simulink model "UAM_Flight_control"  (R2024b)
settings: Solver=FixedStepAuto  StartTime=0.0  StopTime=inf  RelTol=1e-3  EnableMultiTasking=on
undefined symbols (not defined in the file): CityMission, control, controlParams, ControlSampleTime, Cruise_a, DiscIntNeverNeededParam, Earth, FixedWingMission, flightState, FSState, FWControlParams, FWTrimSpeed, HoverMission, params, position, R_WAYPOINTTRANSITION, TransitionMission, uavParam, Vt, w_trim, WGS84, zGround
libraries: slpidlib x56, simulink x35, uavalgslib x8, robotcorelib x2, simulink_extras x2, mspfiltlib x1, aerolibtransform2 x1
(part 11 of 12)

== stateflow chart UAM_Flight_control/Flightmode/Manual/Basic Control  Switching ==
  state STATE_MACHINE
    state Althold
      en:
      flightMode = flightState.Hover;
      %Hover SP
      HoverSPBUS.X = NaN;
      HoverSPBUS.Y = NaN;
      HoverSPBUS.Z = pose(3);
      HoverSPBUS.Yaw = NaN;
    state Stablized
      en:
      flightMode = flightState.Hover;
      %Hover SP
      HoverSPBUS.X = NaN;
      HoverSPBUS.Y = NaN;
      HoverSPBUS.Z = NaN;
      HoverSPBUS.Yaw = NaN;
    state Transition
      en:
      flightMode = flightState.Transition;
      controlMode.inTransition = 1;
      controlMode.TransitionCondition = 0;
    state FWCOMPLETE
      en:
      controlMode.TransitionCondition=1;
      flightMode = flightState.FixedWing;
    state Loiter
      en:
      flightMode = flightState.Hover;
      %Hover SP
      HoverSPBUS.X = pose(1);
      HoverSPBUS.Y = pose(2);
      HoverSPBUS.Z = pose(3);
      HoverSPBUS.Yaw = NaN;
    state Start
      en:
      flightMode=PresetMode;
      %conrtolmode
      controlMode.lateralGuidance = 0;
      controlMode.airspeedAltitude = 0;
      controlMode.attitude = 0;
      controlMode.manual = 1;
      controlMode.armed = 0;
      controlMode.inTransition = 0;
      controlMode.TransitionCondition = 0;
      controlMode.BackTransitionCondition = 0;
      controlMode.land=1;
    state FixedWing
      en:
      flightMode = flightState.FixedWing;
      controlMode.attitude = 1;
      controlMode.inTransition = 0;
      controlMode.TransitionCondition = 1;
    state BackTransition
      en:
      flightMode = flightState.BackTransition;
      controlMode.inTransition = 1;
      controlMode.BackTransitionCondition = 0;
    state HVCOMPLETE
      en:
      controlMode.inTransition = 0;
      controlMode.BackTransitionCondition = 1;
      flightMode = flightState.Hover;
    Stablized -> Althold [order 1] : [trigger(5) >= 1300 && trigger(5) < 1700&& flightMode == flightState.Hover ]
    Althold -> Stablized [order 1] : [trigger(5) < 1300&& flightMode == flightState.Hover ]
    Althold -> Loiter [order 2] : [trigger(5) >= 1700&& flightMode == flightState.Hover ]
    Loiter -> Althold [order 1] : [trigger(5) >= 1300 && trigger(5) < 1700&& flightMode == flightState.Hover ]
    Stablized -> Transition [order 3] : [trigger(7) >=1500 && flightMode == flightState.Hover ]
    Transition -> FWCOMPLETE : [transitionConditionMet(a, Vt)]
    (junction 54) -> Stablized [order 1] : [trigger(7) < 1500 && flightMode == flightState.Hover ]
    (default) -> Start
    Loiter -> Stablized [order 2] : [trigger(5) < 1300&& flightMode == flightState.Hover ]
    Stablized -> Loiter [order 2] : [trigger(5) > 1700&& flightMode == flightState.Hover ]
    Start -> (junction 54)
    (junction 54) -> FixedWing [order 2] : [trigger(7) >= 1500 && flightMode == flightState.FixedWing]
    FixedWing -> BackTransition : [trigger(7) < 15000 && flightMode == flightState.FixedWing]
    BackTransition -> HVCOMPLETE : [backConditionMet(a, States)]
  data: alpha function_input double size=1; valid function_output; Vtransition function_input; alpha function_input; states function_input Bus: GuidanceStates; valid function_output; HoverSPBUS output Bus: HoverSPBus; controlMode output Bus: controlMode; PresetMode input; pose input; States input; trigger input; Vt parameter double; a input size=1; flightMode output
  function valid = transitionConditionMet(alpha, Vtransition):
    | %function valid=transitionConditionMet(TransitionStates,Vtransition)
    | %wingsLevel
    | %if((States.Tilt>=1.57)&&(vecnorm(States.Ve)>Vt))
    | %   valid=true;
    | %else
    | %    valid=false;
    | %end
    | %end
    | 
    | function valid = transitionConditionMet(alpha, Vtransition)
    |     if (alpha >= 1.0) && (vecnorm(States.Ve) > Vtransition)
    |         valid = true;
    |     else
    |         valid = false;
    |     end
    | end
  function valid = backConditionMet(alpha, states):
    | function valid = backConditionMet(alpha, states)
    |     if ( alpha <= 0.01 ) && ( abs(states.Ve(1)) < 4.0 )
    |         valid = true;
    |     else
    |         valid = false;
    |     end
    | end

== matlab function UAM_Flight_control/Controller/Auto1/Fixed Wing Controller/Subsystem/Attitude Controller/Pitch Roll Controller/Turn Coordinator/MATLAB Function ==
  data: rollSP input; rSP output; pitchSP input; airSpeed input
function rSP = fcn(rollSP, pitchSP, airSpeed)
    yawRateSP = tan(rollSP)*9.81/max(airSpeed,5);
    rSP = yawRateSP*cos(pitchSP)*cos(rollSP);
end

== matlab function UAM_Flight_control/Controller/Auto1/Fixed Wing Controller/Subsystem/Lateral Guidance Logic/MATLAB Function ==
  data: courseSP input; lacc output; course input; rollSP output; groundSpeed input; L1 input
function [lacc, rollSP] = fcn(courseSP, course, groundSpeed, L1)
eta = courseSP - course;

% wrap -pi to pi
eta = mod(eta, 2*pi);
if eta>pi
    eta = eta - 2*pi;
end

% cap eta to -pi/2 to pi/2
eta = min(eta, pi/2);
eta = max(eta, -pi/2);

lacc = 2*(groundSpeed^2)/L1*sin(eta);

rollSP = atan(lacc/9.81);

== matlab function UAM_Flight_control/Controller/Auto1/Fixed Wing Controller/Subsystem/Subsystem2/MATLAB Function ==
  data: phi input; y output; theta input
function y = fcn(phi,theta)

y=zeros(3,3);
y=[1 sin(phi)*tan(theta) cos(phi)*tan(theta); 0 cos(phi) -sin(phi); 0 sin(phi)/cos(theta) cos(phi)/cos(theta)];
end

== matlab function UAM_Flight_control/Controller/Emergency/FixedWing Controller/Subsystem/Attitude Controller/Pitch Roll Controller/Turn Coordinator/MATLAB Function ==
  data: rollSP input; rSP output; pitchSP input; airSpeed input
function rSP = fcn(rollSP, pitchSP, airSpeed)
    yawRateSP = tan(rollSP)*9.81/max(airSpeed,5);
    rSP = yawRateSP*cos(pitchSP)*cos(rollSP);
end

== matlab function UAM_Flight_control/Controller/Emergency/FixedWing Controller/Subsystem/Subsystem2/MATLAB Function ==
  data: phi input; y output; theta input
function y = fcn(phi,theta)

y=zeros(3,3);
y=[1 sin(phi)*tan(theta) cos(phi)*tan(theta); 0 cos(phi) -sin(phi); 0 sin(phi)/cos(theta) cos(phi)/cos(theta)];
end

== matlab function UAM_Flight_control/Controller/Manual/FixedWing Controller/Subsystem/Attitude Controller/Pitch Roll Controller/Turn Coordinator/MATLAB Function ==
  data: rollSP input; rSP output; pitchSP input; airSpeed input
function rSP = fcn(rollSP, pitchSP, airSpeed)
    yawRateSP = tan(rollSP)*9.81/max(airSpeed,5);
    rSP = yawRateSP*cos(pitchSP)*cos(rollSP);
end

== matlab function UAM_Flight_control/Controller/Manual/FixedWing Controller/Subsystem/Subsystem2/MATLAB Function ==
  data: phi input; y output; theta input
function y = fcn(phi,theta)

y=zeros(3,3);
y=[1 sin(phi)*tan(theta) cos(phi)*tan(theta); 0 cos(phi) -sin(phi); 0 sin(phi)/cos(theta) cos(phi)/cos(theta)];
end

== matlab function UAM_Flight_control/Controller/Manual/multicopter Controller/Attitude & Altitude controller/Derivative Gain/deadzone/MATLAB Function ==
  data: trigger input; yaw_sp output; euler_yaw input
function yaw_sp = yaw_hold(trigger, euler_yaw)
persistent last_yaw_sp

if isempty(last_yaw_sp)
    last_yaw_sp = 0;
end

if trigger == 1
    last_yaw_sp = euler_yaw;
end

yaw_sp = last_yaw_sp;

== matlab function UAM_Flight_control/Controller/Manual/Scheduler/Subsystem/Switch Case Action Subsystem/Desaturation ==
  data: m_in input; m_out output; mixMat input
%{
function m_out = desat_px4(m_in, mixMat)

% PX4-style desaturation (Stabilized, MC_AIRMODE=0, 튜닝용)

m = m_in(:);
[N, cols] = size(mixMat);
assert(numel(m)==N && cols==4, 'mixMat must be [Nm x 4]');

act_min = zeros(N,1);
act_max = ones(N,1);
MINIMUM_YAW_MARGIN = 0.15;

thrust_z = mixMat(:,1);
roll_vec = mixMat(:,2);
pitch_vec= mixMat(:,3);
yaw_vec  = mixMat(:,4);

% 1) thrust axis (thrust can only decrease)
m = desat_axis(m, thrust_z, act_min, act_max, true);

% 2) roll/pitch torques
m = desat_axis(m, roll_vec, act_min, act_max, false);
m = desat_axis(m, pitch_vec, act_min, act_max, false);

% 3) yaw with margin
act_max_yaw = act_max + (act_max - act_min) * MINIMUM_YAW_MARGIN;
m = desat_axis(m, yaw_vec, act_min, act_max_yaw, false);

% thrust again (only down)
m = desat_axis(m, thrust_z, act_min, act_max, true);

m_out = max(act_min, min(act_max, m));
end

function m = desat_axis(m, dir, act_min, act_max, thrust_only_down)
    k = compute_gain(dir, m, act_min, act_max);
    if ~(thrust_only_down && k > 0)
        m = m + k * dir;
    end

    k = 0.5 * compute_gain(dir, m, act_min, act_max);
    if ~(thrust_only_down && k > 0)
        m = m + k * dir;
    end
end

function k = compute_gain(dir, m, act_min, act_max)
    k_min = 0.0; 
    k_max = 0.0;

    for i = 1:numel(m)
        if abs(dir(i)) < 0.2
            continue;
        end

        if m(i) < act_min(i)
            ki = (act_min(i) - m(i)) / dir(i);
            k_min = min(k_min, ki);
            k_max = max(k_max, ki);
        end

        if m(i) > act_max(i)
            ki = (act_max(i) - m(i)) / dir(i);
            k_min = min(k_min, ki);
            k_max = max(k_max, ki);
        end
    end

    k = k_min + k_max;
end
%}

function m_out = desat_px4(m_in, mixMat)
% PX4-style desaturation (MC_AIRMODE = 1, Roll/Pitch airmode)

m = m_in(:);
[N, cols] = size(mixMat);
assert(numel(m)==N && cols==4, 'mixMat must be [Nm x 4]');

act_min = zeros(N,1);
act_max = ones(N,1);
MINIMUM_YAW_MARGIN = 0.15;

thrust_z = mixMat(:,1);
roll_vec  = mixMat(:,2); %#ok<NASGU>
pitch_vec = mixMat(:,3); %#ok<NASGU>
yaw_vec   = mixMat(:,4);

% 1) thrust axis (airmode: up/down 둘 다 허용)
m = desat_axis(m, thrust_z, act_min, act_max, false);

% 2) roll/pitch는 따로 줄이지 않음 (RP airmode: 자세 우선)

% 3) yaw with margin (mixYaw()와 동일 개념)
act_max_yaw = act_max + (act_max - act_min) * MINIMUM_YAW_MARGIN;
m = desat_axis(m, yaw_vec, act_min, act_max_yaw, false);

% 4) thrust again (only down, 0~1 안으로)
m = desat_axis(m, thrust_z, act_min, act_max, true);

m_out = max(act_min, min(act_max, m));
end

function m = desat_axis(m, dir, act_min, act_max, thrust_only_down)
    k = compute_gain(dir, m, act_min, act_max);
    if ~(thrust_only_down && k > 0)
        m = m + k * dir;
    end

    k = 0.5 * compute_gain(dir, m, act_min, act_max);
    if ~(thrust_only_down && k > 0)
        m = m + k * dir;
    end
end

function k = compute_gain(dir, m, act_min, act_max)
    k_min = 0.0;
    k_max = 0.0;

    for i = 1:numel(m)
        if abs(dir(i)) < 0.2
            continue;
        end

        if m(i) < act_min(i)
            ki = (act_min(i) - m(i)) / dir(i);
            k_min = min(k_min, ki);
            k_max = max(k_max, ki);
        end

        if m(i) > act_max(i)
            ki = (act_max(i) - m(i)) / dir(i);
            k_min = min(k_min, ki);
            k_max = max(k_max, ki);
        end
    end

    k = k_min + k_max;
end

== matlab function UAM_Flight_control/Controller/Manual/multicopter Controller/Attitude & Altitude controller/Derivative Gain/MATLAB Function ==
  data: x input; y output
function y = wrapToPi(x)
% x : angle error (rad)
% y : wrapped to [-pi, pi]
y = atan2(sin(x), cos(x));

== matlab function UAM_Flight_control/Controller/Manual/multicopter Controller/Atitude Control/MATLAB Function ==
  data: x input; y output
function y = wrapToPi(x)
% x : angle error (rad)
% y : wrapped to [-pi, pi]
y = atan2(sin(x), cos(x));

== matlab function UAM_Flight_control/Controller/Manual/multicopter Controller/Atitude Control/deadzone/MATLAB Function ==
  data: trigger input; yaw_sp output; euler_yaw input
function yaw_sp = yaw_hold(trigger, euler_yaw)
persistent last_yaw_sp

if isempty(last_yaw_sp)
    last_yaw_sp = 0;
end

if trigger == 1
    last_yaw_sp = euler_yaw;
end

yaw_sp = last_yaw_sp;

== matlab function UAM_Flight_control/Sensor/MATLAB Function ==
  data: pressure_kPa input; P0_Pa output; arm input; valid output
function [P0_Pa, valid] = latch_pressure_kPa(pressure_kPa, arm)
%#codegen
% Latch P0 at ARM rising edge (arm: 0 -> 1)

persistent p0_set p0_Pa last_arm
if isempty(p0_set)
    p0_set   = false;
    p0_Pa    = 0.0;
    last_arm = uint8(0);
end

P_Pa   = pressure_kPa * 1000.0;
arm_u8 = uint8(arm ~= 0);

% ---- Detect arm edge ----
arm_rising = (last_arm == 0) && (arm_u8 == 1);
arm_falling = (last_arm == 1) && (arm_u8 == 0);

% ---- ARM rising edge: latch P0 ----
if arm_rising
    if isfinite(P_Pa) && P_Pa > 0
        p0_Pa  = P_Pa;
        p0_set = true;
    else
        p0_Pa  = 0.0;
        p0_set = false;
    end
end

% ---- ARM falling edge: reset ----
if arm_falling
    p0_set = false;
    p0_Pa  = 0.0;
end

last_arm = arm_u8;

% ---- Outputs ----
P0_Pa = p0_Pa;
valid = p0_set;
end

== matlab function UAM_Flight_control/Sensor/Subsystem1/Subsystem/MATLAB Function1 ==
  data: theta input; dq output
function dq = dq_from_theta(theta)
%#codegen
% theta: 3x1 = 0.5*(w-bg)*dt  (half-angle already applied)
% dq   : 4x1 quaternion increment [w;x;y;z]

a = sqrt(theta(1)^2 + theta(2)^2 + theta(3)^2);

if a < 1e-8
    % small-angle: sin(a)/a ≈ 1, cos(a) ≈ 1
    dq = [1.0;
          theta(1);
          theta(2);
          theta(3)];
else
    s = sin(a) / a;
    dq = [cos(a);
          theta(1)*s;
          theta(2)*s;
          theta(3)*s];
end
end

== matlab function UAM_Flight_control/Sensor/Subsystem1/Subsystem/MATLAB Function2 ==
  data: q input; qout output; dq input
function qout = quat_mul(q, dq)
%#codegen
% qout = q ⊗ dq, both [w;x;y;z]
w1=q(1); x1=q(2); y1=q(3); z1=q(4);
w2=dq(1); x2=dq(2); y2=dq(3); z2=dq(4);

qout = [ w1*w2 - x1*x2 - y1*y2 - z1*z2;
         w1*x2 + x1*w2 + y1*z2 - z1*y2;
         w1*y2 - x1*z2 + y1*w2 + z1*x2;
         w1*z2 + x1*y2 - y1*x2 + z1*w2 ];
end

== matlab function UAM_Flight_control/Sensor/Subsystem1/Subsystem/normalize ==
  data: q input; qn output
function qn = quat_norm(q)
%#codegen
n = sqrt(q(1)^2 + q(2)^2 + q(3)^2 + q(4)^2);
if n > 0
    qn = q / n;
else
    qn = [1;0;0;0];
end
end

== matlab function UAM_Flight_control/Sensor/Subsystem1/MATLAB Function1 ==
  data: q input; R output
function R = quat_to_R_bn(q)
%#codegen
% q: [w; x; y; z] (unit quaternion)
% R: Body -> NED rotation matrix

w = q(1); x = q(2); y = q(3); z = q(4);

% Precompute products
ww = w*w; xx = x*x; yy = y*y; zz = z*z;

R = zeros(3,3);

R(1,1) = ww + xx - yy - zz;
R(1,2) = 2*(x*y - w*z);
R(1,3) = 2*(x*z + w*y);

R(2,1) = 2*(x*y + w*z);
R(2,2) = ww - xx + yy - zz;
R(2,3) = 2*(y*z - w*x);

R(3,1) = 2*(x*z - w*y);
R(3,2) = 2*(y*z + w*x);
R(3,3) = ww - xx - yy + zz;
end

== matlab function UAM_Flight_control/Sensor/MATLAB Function2 ==
  data: pressure_kPa input; z_baro output; P0_Pa input; P0_valid input
function z_baro = baro_z_from_pressure(pressure_kPa, P0_Pa, P0_valid)
%#codegen

% 입력 압력 (Pa)
P = pressure_kPa * 1000.0;

if ~P0_valid || P0_Pa <= 0
    z_baro = 0.0;
    return;
end

% ---- 고도 계산: P는 래치된 값 사용 ----
ratio = P / P0_Pa;
h_up  = 44330.0 * (1.0 - ratio.^0.1903); % Up(+), m
z_baro = -h_up;                         % NED Down(+)
end

== matlab function UAM_Flight_control/Sensor/Subsystem1/MATLAB Function3 ==
  data: Pzz input; Pzz_n output; Pzv input; Pvv input; dt input; Qzz input; Qvv input; Pzv_n output; Pvv_n output
function [Pzz_n, Pzv_n, Pvv_n] = cov_predict(Pzz, Pzv, Pvv, dt, Qzz, Qvv)
%#codegen

Pzz_n = Pzz + 2*dt*Pzv + dt*dt*Pvv + Qzz;
Pzv_n = Pzv + dt*Pvv;
Pvv_n = Pvv + Qvv;

end

== matlab function UAM_Flight_control/Sensor/Subsystem1/MATLAB Function4 ==
  data: gps_h_msl input; z_gps_ned output; ref_valid output
function [z_gps_ned, ref_valid] = latch_gps_z_firstvalid(gps_h_msl)
%#codegen
% gps_h_msl : GNSS absolute altitude (m, Up+). Some systems output 0 when invalid.
% z_gps_ned : relative altitude in NED Down(+) [m] (up -> negative)
% ref_valid : reference latched?

persistent ref_set h_ref last_z
if isempty(ref_set)
    ref_set = false;
    h_ref   = 0.0;
    last_z  = 0.0;
end

% ---- define validity check ----
% Treat non-finite or near-zero as invalid (tune threshold if your system can be near sea level).
is_valid = isfinite(gps_h_msl) && (abs(gps_h_msl) > 1.0);

% ---- latch reference on first valid sample ----
if ~ref_set && is_valid
    h_ref   = gps_h_msl;
    ref_set = true;
end

% ---- output ----
if ref_set && is_valid
    z_gps_ned = -(gps_h_msl - h_ref);
    last_z    = z_gps_ned;   % optional: hold last good output
    ref_valid = true;
else
    % If reference not ready or GPS temporarily invalid:
    z_gps_ned = last_z;      % hold last value (or 0.0 if you prefer)
    ref_valid = ref_set;     % true if we already latched ref at least once
end
end

== matlab function UAM_Flight_control/Sensor/MATLAB Function5 ==
  data: z_in input; z_lpf output; P0_valid input; valid output
function [z_lpf, valid] = lpf_z_baro(z_in, P0_valid)
%#codegen
% 1st-order discrete LPF:
%   y[k] = y[k-1] + alpha*(x[k] - y[k-1])
%
% Inputs:
%   z_in     : raw z_baro (m, NED Down +)
%   P0_valid : 0/1 (baro reference valid)
%
% Outputs:
%   z_lpf  : filtered z_baro
%   valid  : filtered output valid (same as P0_valid)

persistent y init
if isempty(init)
    y = 0.0;
    init = false;
end

% ---- Parameters (SET THESE) ----
Ts = 0.005;     % sample time [s] (200 Hz -> 0.005)
fc = 1.0;       % cutoff [Hz] (try 0.5~2.0)

% alpha = 1 - exp(-2*pi*fc*Ts)
alpha = 1.0 - exp(-2.0*pi*fc*Ts);

% ---- Valid handling ----
valid = (P0_valid ~= 0);

if ~valid || ~isfinite(z_in)
    % reset state when reference invalid
    y = 0.0;
    init = false;
    z_lpf = 0.0;
    return;
end

% ---- Initialize output to first input to avoid big transient ----
if ~init
    y = z_in;
    init = true;
    z_lpf = y;
    return;
end

% ---- LPF update ----
y = y + alpha*(z_in - y);
z_lpf = y;
end

== matlab function UAM_Flight_control/Controller/Manual/multicopter Controller/Altitude Control1/Normalization( -1 ~ 1)/MATLAB Function ==
  data: u input; y output; expo input
 function y = expo_curve(u, expo)                                                                                               
  % PX4 Exponential Curve                                                                                                        
  % u    : 입력 (-1 ~ 1 범위, Dead Zone 통과 후 정규화된 스틱 값)                                                                
  % expo : Expo 계수 (0 = 선형, 1 = 완전 큐빅, PX4 기본값 0.6)                                                                   
  % y    : 출력 (-1 ~ 1 범위)                                                                                                    
                                                                                                                                 
  y = sign(u) * (expo * abs(u)^3 + (1 - expo) * abs(u));                                                                         
                                                                                                                                 
  end

== matlab function UAM_Flight_control/Controller/Manual/multicopter Controller/Altitude Control1/MATLAB Function ==
  data: thrust_in input; vz input; az input; hover_est output; active input
  function hover_est = hover_thrust_lpf(thrust_in, vz, az, active)                                                  
      %#codegen                                            
      persistent hover_thrust                              
                                                           
      % Constants                                          
      HOVER_MIN = 0.2;                                     
      HOVER_MAX = 0.8;                                     
      SLEW_RATE = 0.0005;  % 200Hz 기준, 초당 0.1 변화     
      GRAVITY = 9.81;                                      
                                                           
      % Thresholds                                         
      VZ_LIM = 0.5;   % m/s                                
      AZ_LIM = 1.0;   % m/s²                               
                                                           
      if isempty(hover_thrust)                             
          hover_thrust = 0.5;                              
      end                                                  
                                                           
      hover_est = hover_thrust;                            
                                                           
      % 중력 제거                                          
      az_compensated = az + GRAVITY;                       
                                                           
      % 안정 조건 체크                                     
      is_stable = (abs(vz) < VZ_LIM) && (abs(az_compensated) < AZ_LIM);                          
                                                           
      if active && is_stable                               
          err = thrust_in - hover_thrust;                  
                                                           
          if err > SLEW_RATE                               
              hover_thrust = hover_thrust + SLEW_RATE;     
          elseif err < -SLEW_RATE                          
              hover_thrust = hover_thrust - SLEW_RATE;     
          else                                             
              hover_thrust = thrust_in;                    
          end                                              
                                                           
          hover_thrust = max(HOVER_MIN, min(HOVER_MAX, hover_thrust));                                          
      end                                                  
  end

== matlab function UAM_Flight_control/Sensor/MATLAB Function8 ==
  data: raw_acc input; pos_out output; raw_gyro input; raw_gps_lat input; raw_gps_lon input; raw_gps_alt input; raw_gps_vel input; baro_alt input; mag input; quat_prev input; vel_prev input; pos_prev input; gyro_bias_prev input; accel_bias_prev input; P_prev input; baro_bias_prev input; dt input; ref_lat input; ref_lon input; ref_alt input; gps_valid input; baro_valid input; vel_out output; quat_out output; gyro_bias_out output; accel_bias_out output; pos_var_out output; vel_var_out output; P_out output; baro_bias_out output
 function [pos_out, vel_out, quat_out, gyro_bias_out, accel_bias_out, ...  
            pos_var_out, vel_var_out, P_out, baro_bias_out] = ...                                                                                                               
      EKF2_Main(raw_acc, raw_gyro, raw_gps_lat, raw_gps_lon, raw_gps_alt, raw_gps_vel, ...
                baro_alt, mag, ...                                                                                                                                              
                quat_prev, vel_prev, pos_prev, gyro_bias_prev, accel_bias_prev, ...                                                                                             
                P_prev, baro_bias_prev, dt, ref_lat, ref_lon, ref_alt, ...                                                                                                      
                gps_valid, baro_valid)
  %% ================================================================
  %% PX4 EKF2 Style Extended Kalman Filter - VN-300 Raw Data Version
  %% GPS fusion distributed: 1 measurement per step (no timing overrun)
  %% ================================================================

  %% Parameters
  EKF2_GYR_NOISE   = 0.0035;
  EKF2_ACC_NOISE   = 0.14;
  EKF2_GYR_B_NOISE = 0.0001;
  EKF2_ACC_B_NOISE = 0.005;

  EKF2_BARO_NOISE    = 1.5;
  EKF2_GPS_P_NOISE   = 2.5;
  EKF2_GPS_V_NOISE   = 0.5;
  EKF2_GPS_ALT_NOISE = 5.0;

  INNOV_GATE = 5.0;
  g = 9.81;

  %% Initialize outputs
  quat_out       = zeros(4, 1);
  vel_out        = zeros(3, 1);
  pos_out        = zeros(3, 1);
  gyro_bias_out  = zeros(3, 1);
  accel_bias_out = zeros(3, 1);
  pos_var_out    = zeros(3, 1);
  vel_var_out    = zeros(3, 1);
  P_out          = zeros(24, 24);
  baro_bias_out  = 0;

  quat_out       = quat_prev;
  vel_out        = vel_prev;
  pos_out        = pos_prev;
  gyro_bias_out  = gyro_bias_prev;
  accel_bias_out = accel_bias_prev;
  P_out          = P_prev;
  baro_bias_out  = baro_bias_prev;

  %% GPS fusion round-robin counter
  persistent fuse_idx
  if isempty(fuse_idx)
      fuse_idx = uint8(0);
  end

  %% ========== 0. Quaternion safety check ==========
  nq = norm(quat_prev);
  if nq < 1e-10
      quat_prev = [1; 0; 0; 0];
  else
      quat_prev = quat_prev / nq;
  end

  %% ========== 1. State Prediction ==========
  gyro_corrected = raw_gyro - gyro_bias_prev;
  acc_corrected  = raw_acc  - accel_bias_prev;

  q = quat_prev;
  omega = gyro_corrected;

  q_dot = 0.5 * [0, -omega(1), -omega(2), -omega(3);
                 omega(1), 0, omega(3), -omega(2);
                 omega(2), -omega(3), 0, omega(1);
                 omega(3), omega(2), -omega(1), 0] * q;

  quat_pred = q + q_dot * dt;
  n = norm(quat_pred);
  if n < 1e-10
      quat_pred = [1; 0; 0; 0];
  else
      quat_pred = quat_pred / n;
  end

  q0 = quat_pred(1); q1 = quat_pred(2); q2 = quat_pred(3); q3 = quat_pred(4);
  R_bn = [q0^2+q1^2-q2^2-q3^2, 2*(q1*q2-q0*q3), 2*(q1*q3+q0*q2);
          2*(q1*q2+q0*q3), q0^2-q1^2+q2^2-q3^2, 2*(q2*q3-q0*q1);
          2*(q1*q3-q0*q2), 2*(q2*q3+q0*q1), q0^2-q1^2-q2^2+q3^2];

  acc_ned = R_bn * acc_corrected;
  vel_pred = vel_prev + (acc_ned + [0; 0; g]) * dt;
  pos_pred = pos_prev + vel_prev * dt + 0.5 * (acc_ned + [0; 0; g]) * dt^2;

  %% ========== 2. Covariance Prediction ==========
  Q = zeros(24, 24);
  Q(1:3, 1:3)     = eye(3) * EKF2_GYR_NOISE^2 * dt^2;
  Q(4:6, 4:6)     = eye(3) * EKF2_ACC_NOISE^2 * dt^2;
  Q(7:9, 7:9)     = eye(3) * EKF2_ACC_NOISE^2 * dt^4/4;
  Q(10:12, 10:12) = eye(3) * EKF2_GYR_B_NOISE^2 * dt^2;
  Q(13:15, 13:15) = eye(3) * EKF2_ACC_B_NOISE^2 * dt^2;

  F = eye(24);
  F(4:6, 1:3)   = -R_bn * skew(acc_corrected) * dt;
  F(7:9, 4:6)   = eye(3) * dt;
  F(4:6, 13:15) = -R_bn * dt;
  F(1:3, 10:12) = -eye(3) * dt;

  P_pred = F * P_prev * F' + Q;

  %% ========== 3. Measurement Updates ==========

  %% 3.1 Barometer Height Fusion (매 스텝)
  if baro_valid
      R_baro = EKF2_BARO_NOISE^2;
      H_baro = zeros(1, 24);
      H_baro(9) = 1;

      z_baro = -(baro_alt - ref_alt) - baro_bias_prev;
      innov_baro = z_baro - pos_pred(3);
      innov_var_baro = H_baro * P_pred * H_baro' + R_baro;

      if abs(innov_baro) < INNOV_GATE * sqrt(innov_var_baro)
          K_baro = P_pred * H_baro' / innov_var_baro;
          dx = K_baro * innov_baro;

          dq = [1; 0.5*dx(1:3)];
          quat_pred = quatmul(dq, quat_pred);
          quat_pred = quat_pred / norm(quat_pred);

          vel_pred = vel_pred + dx(4:6);
          pos_pred = pos_pred + dx(7:9);
          gyro_bias_prev  = gyro_bias_prev  + dx(10:12);
          accel_bias_prev = accel_bias_prev + dx(13:15);

          IKH = eye(24) - K_baro * H_baro;
          P_pred = IKH * P_pred * IKH' + K_baro * R_baro * K_baro';
      end
  end

  %% 3.2 GPS Fusion: 스텝당 1개씩 round-robin (N,E,D,vN,vE,vD)
  if gps_valid
      Re = 6378137.0;
      lat_rad = ref_lat * pi / 180;
      dN = (raw_gps_lat - ref_lat) * pi / 180 * Re;
      dE = (raw_gps_lon - ref_lon) * pi / 180 * Re * cos(lat_rad);
      dD = -(raw_gps_alt - ref_alt);

      fuse_idx = fuse_idx + uint8(1);
      if fuse_idx > uint8(6)
          fuse_idx = uint8(1);
      end

      H_gps = zeros(1, 24);
      innov_gps = 0;
      R_gps = 0;

      switch fuse_idx
          case uint8(1)  %% GPS North position
              H_gps(7) = 1;
              innov_gps = dN - pos_pred(1);
              R_gps = EKF2_GPS_P_NOISE^2;
          case uint8(2)  %% GPS East position
              H_gps(8) = 1;
              innov_gps = dE - pos_pred(2);
              R_gps = EKF2_GPS_P_NOISE^2;
          case uint8(3)  %% GPS Down position
              H_gps(9) = 1;
              innov_gps = dD - pos_pred(3);
              R_gps = EKF2_GPS_ALT_NOISE^2;
          case uint8(4)  %% GPS North velocity
              H_gps(4) = 1;
              innov_gps = raw_gps_vel(1) - vel_pred(1);
              R_gps = EKF2_GPS_V_NOISE^2;
          case uint8(5)  %% GPS East velocity
              H_gps(5) = 1;
              innov_gps = raw_gps_vel(2) - vel_pred(2);
              R_gps = EKF2_GPS_V_NOISE^2;
          case uint8(6)  %% GPS Down velocity
              H_gps(6) = 1;
              innov_gps = raw_gps_vel(3) - vel_pred(3);
              R_gps = EKF2_GPS_V_NOISE^2;
      end

      innov_var_gps = H_gps * P_pred * H_gps' + R_gps;

      if abs(innov_gps) < INNOV_GATE * sqrt(innov_var_gps)
          K_gps = P_pred * H_gps' / innov_var_gps;
          dx = K_gps * innov_gps;

          dq = [1; 0.5*dx(1:3)];
          quat_pred = quatmul(dq, quat_pred);
          quat_pred = quat_pred / norm(quat_pred);

          vel_pred = vel_pred + dx(4:6);
          pos_pred = pos_pred + dx(7:9);
          gyro_bias_prev  = gyro_bias_prev  + dx(10:12);
          accel_bias_prev = accel_bias_prev + dx(13:15);

          IKH = eye(24) - K_gps * H_gps;
          P_pred = IKH * P_pred * IKH' + K_gps * R_gps * K_gps';
      end
  else
      fuse_idx = uint8(0);  %% GPS 끊기면 리셋
  end

  %% ========== 4. Baro Bias Estimation ==========
  if baro_valid
      alpha_baro = 0.01;
      baro_meas = -(baro_alt - ref_alt);
      baro_bias_out = baro_bias_prev + alpha_baro * (baro_meas + pos_pred(3) - baro_bias_prev);
  else
      baro_bias_out = baro_bias_prev;
  end

  %% ========== 5. Output ==========
  quat_out       = quat_pred;
  vel_out        = vel_pred;
  pos_out        = pos_pred;
  gyro_bias_out  = gyro_bias_prev;
  accel_bias_out = accel_bias_prev;
  P_out          = P_pred;

  pos_var_out = [P_out(7,7); P_out(8,8); P_out(9,9)];
  vel_var_out = [P_out(4,4); P_out(5,5); P_out(6,6)];

  end

  %% ========== Helper: Quaternion multiplication ==========
  function qout = quatmul(a, b)
      qout = [a(1)*b(1) - a(2)*b(2) - a(3)*b(3) - a(4)*b(4);
              a(1)*b(2) + a(2)*b(1) + a(3)*b(4) - a(4)*b(3);
              a(1)*b(3) - a(2)*b(4) + a(3)*b(1) + a(4)*b(2);
              a(1)*b(4) + a(2)*b(3) - a(3)*b(2) + a(4)*b(1)];
  end

  %% ========== Helper: Skew-symmetric matrix ==========
  function S = skew(v)
      S = [0, -v(3), v(2);
           v(3), 0, -v(1);
           -v(2), v(1), 0];
  end

== matlab function UAM_Flight_control/Sensor/MATLAB Function9 ==
  data: raw_gps_lat input; ref_lat output; raw_gps_lon input; raw_gps_alt input; gps_valid input; ref_lon output; ref_alt output
function [ref_lat, ref_lon, ref_alt] = ref_init(raw_gps_lat, raw_gps_lon, raw_gps_alt, gps_valid)
%% GPS Reference Point Latch
%% 첫 번째 유효 GPS 데이터를 NED 좌표계 원점으로 저장하고 이후 고정
%%
%% Inputs:
%%   raw_gps_lat  <- fcc.raw_gps_lat  (degrees)
%%   raw_gps_lon  <- fcc.raw_gps_lon  (degrees)
%%   raw_gps_alt  <- fcc.raw_gps_alt  (m, WGS-84)
%%   gps_valid    <- fcc.gps_valid    (0 or 1)
%%
%% Outputs:
%%   ref_lat, ref_lon, ref_alt -> EKF2_Main 입력으로 연결

persistent lat0 lon0 alt0 locked

if isempty(locked)
    locked = false;
    lat0 = 0;
    lon0 = 0;
    alt0 = 0;
end

if ~locked && gps_valid == 1
    lat0 = raw_gps_lat;
    lon0 = raw_gps_lon;
    alt0 = raw_gps_alt;
    locked = true;
end

ref_lat = lat0;
ref_lon = lon0;
ref_alt = alt0;

end

== matlab function UAM_Flight_control/Controller/Auto1/Multicopter Controller/Attitude & Altitude controller/Altitude Control/MATLAB Function1 ==
  data: thrust_in input; vz input; az input; hover_est output; active input
  function hover_est = hover_thrust_lpf(thrust_in, vz, az, active)                                                  
      %#codegen                                            
      persistent hover_thrust                              
                                                           
      % Constants                                          
      HOVER_MIN = 0.2;                                     
      HOVER_MAX = 0.8;                                     
      SLEW_RATE = 0.0005;  % 200Hz 기준, 초당 0.1 변화     
      GRAVITY = 9.81;                                      
                                                           
      % Thresholds                                         
      VZ_LIM = 0.5;   % m/s                                
      AZ_LIM = 1.0;   % m/s²                               
                                                           
      if isempty(hover_thrust)                             
          hover_thrust = 0.5;                              
      end                                                  
                                                           
      hover_est = hover_thrust;                            
                                                           
      % 중력 제거                                          
      az_compensated = az + GRAVITY;                       
                                                           
      % 안정 조건 체크                                     
      is_stable = (abs(vz) < VZ_LIM) && (abs(az_compensated) < AZ_LIM);                          
                                                           
      if active && is_stable                               
          err = thrust_in - hover_thrust;                  
                                                           
          if err > SLEW_RATE                               
              hover_thrust = hover_thrust + SLEW_RATE;     
          elseif err < -SLEW_RATE                          
              hover_thrust = hover_thrust - SLEW_RATE;     
          else                                             
              hover_thrust = thrust_in;                    
          end                                              
                                                           
          hover_thrust = max(HOVER_MIN, min(HOVER_MAX, hover_thrust));                                          
      end                                                  
  end

== matlab function UAM_Flight_control/Controller/Manual/multicopter Controller/Horizontal Position Control1/MATLAB Function ==
  data: u input; y output; expo input
function y = expo_curve(u, expo)      

    y = sign(u) * (expo * abs(u)^3 + (1 - expo) * abs(u));   
    
end

== matlab function UAM_Flight_control/Controller/Manual/multicopter Controller/Horizontal Position Control1/MATLAB Function1 ==
  data: u input; y output; expo input
function y = expo_curve(u, expo)      

    y = sign(u) * (expo * abs(u)^3 + (1 - expo) * abs(u));   
    
end

== matlab function UAM_Flight_control/Controller/Auto1/Multicopter Controller/Attitude & Altitude controller/Altitude Control/Subsystem/MATLAB Function ==
  data: thrust_in input; vz input; az input; hover_est output; active input
  function hover_est = hover_thrust_lpf(thrust_in, vz, az, active)                                                  
      %#codegen                                            
      persistent hover_thrust                              
                                                           
      % Constants                                          
      HOVER_MIN = 0.2;                                     
      HOVER_MAX = 0.8;                                     
      SLEW_RATE = 0.003;  % 200Hz 기준, 초당 0.1 변화     
      GRAVITY = 9.81;                                      
                                                           
      % Thresholds                                         
      VZ_LIM = 0.5;   % m/s                                
      AZ_LIM = 1.0;   % m/s²                               
                                                           
      if isempty(hover_thrust)                             
          hover_thrust = 0.5;                              
      end                                                  
                                                           
      hover_est = hover_thrust;                            
                                                           
      % 중력 제거                                          
      az_compensated = az + GRAVITY;                       
                                                           
      % 안정 조건 체크                                     
      is_stable = (abs(vz) < VZ_LIM) && (abs(az_compensated) < AZ_LIM);                          
                                                           
      if active && is_stable                               
          err = thrust_in - hover_thrust;                  
                                                           
          if err > SLEW_RATE                               
              hover_thrust = hover_thrust + SLEW_RATE;     
          elseif err < -SLEW_RATE                          
              hover_thrust = hover_thrust - SLEW_RATE;     
          else                                             
              hover_thrust = thrust_in;                    
          end                                              
                                                           
          hover_thrust = max(HOVER_MIN, min(HOVER_MAX, hover_thrust));                                          
      end                                                  
  end

== matlab function UAM_Flight_control/Controller/Auto1/Multicopter Controller/Attitude & Altitude controller/Derivative Gain/MATLAB Function ==
  data: x input; y output
function y = wrapToPi(x)
% x : angle error (rad)
% y : wrapped to [-pi, pi]
y = atan2(sin(x), cos(x));

== matlab function UAM_Flight_control/Controller/Auto1/Scheduler/Subsystem/Switch Case Action Subsystem/Desaturation ==
  data: m_in input; m_out output; mixMat input
function m_out = desat_px4(m_in, mixMat)
% PX4-style desaturation (MC_AIRMODE = 1, Roll/Pitch airmode)

m = m_in(:);
[N, cols] = size(mixMat);
assert(numel(m)==N && cols==4, 'mixMat must be [Nm x 4]');

act_min = zeros(N,1);
act_max = ones(N,1);
MINIMUM_YAW_MARGIN = 0.15;

thrust_z = mixMat(:,1);
roll_vec  = mixMat(:,2); %#ok<NASGU>
pitch_vec = mixMat(:,3); %#ok<NASGU>
yaw_vec   = mixMat(:,4);

% 1) thrust axis (airmode: up/down 둘 다 허용)
m = desat_axis(m, thrust_z, act_min, act_max, false);

% 2) roll/pitch는 따로 줄이지 않음 (RP airmode: 자세 우선)

% 3) yaw with margin (mixYaw()와 동일 개념)
act_max_yaw = act_max + (act_max - act_min) * MINIMUM_YAW_MARGIN;
m = desat_axis(m, yaw_vec, act_min, act_max_yaw, false);

% 4) thrust again (only down, 0~1 안으로)
m = desat_axis(m, thrust_z, act_min, act_max, true);

m_out = max(act_min, min(act_max, m));
end

function m = desat_axis(m, dir, act_min, act_max, thrust_only_down)
    k = compute_gain(dir, m, act_min, act_max);
    if ~(thrust_only_down && k > 0)
        m = m + k * dir;
    end

    k = 0.5 * compute_gain(dir, m, act_min, act_max);
    if ~(thrust_only_down && k > 0)
        m = m + k * dir;
    end
end

function k = compute_gain(dir, m, act_min, act_max)
    k_min = 0.0;
    k_max = 0.0;

    for i = 1:numel(m)
        if abs(dir(i)) < 0.2
            continue;
        end

        if m(i) < act_min(i)
            ki = (act_min(i) - m(i)) / dir(i);
            k_min = min(k_min, ki);
            k_max = max(k_max, ki);
        end

        if m(i) > act_max(i)
            ki = (act_max(i) - m(i)) / dir(i);
            k_min = min(k_min, ki);
            k_max = max(k_max, ki);
        end
    end

    k = k_min + k_max;
end

== matlab function UAM_Flight_control/Sensor/MATLAB Function6 ==
  data: YPR_raw input; YPR_corrected output; arm input
function YPR_corrected = IMU_Bias_Correction(YPR_raw, arm)
%#codegen

% Persistent variable to store bias
persistent ypr_bias;
persistent armed_prev;

if isempty(ypr_bias)
    ypr_bias = zeros(3,1);
    armed_prev = 0;
end

% Capture bias on rising edge of arm signal
if arm >= 1 && armed_prev < 1
    ypr_bias = YPR_raw;
end

armed_prev = arm;

% Apply bias correction
YPR_corrected = YPR_raw - ypr_bias;

== matlab function UAM_Flight_control/Flightmode/Auto/Guidance Mode Selector/GuidanceLogic.Land.Descend/MATLAB Function ==
  data: FromWP input Bus: UAVPathManagerBus size=1; wps output; ToWPPos input size=[3 1]; ToWPParam input size=[4 1]
function wps = getLandingWaypoint(FromWP, ToWPPos, ToWPParam)

persistent outWPS

if isempty(outWPS)
    outWPS = double(zeros(2,4));
end

outWPS(1,:) = [FromWP.position' FromWP.params(1)];
outWPS(2,:) = [reshape(ToWPPos,1,[]), ToWPParam(1)];

wps = outWPS;

== matlab function UAM_Flight_control/Flightmode/Auto/Guidance Mode Selector/GuidanceLogic.Land.Descend/MATLAB Function1 ==
  data: current_alt input; descent_speed output; land_alt input
function descent_speed = calcDescentSpeed(current_alt, land_alt)
      % 지면 위 고도 (AGL)
      dist_to_ground = abs(current_alt - land_alt);

      % PX4 스타일 파라미터
      LAND_ALT1 = 10.0;    % 감속 시작 고도 (m)
      LAND_ALT2 = 5.0;     % 저속 도달 고도 (m)
      LAND_ALT3 = 1.0;     % 극저속 전환 고도 (m)
      CRUISE_DN = 2.0;     % 고고도 하강 속도 (m/s)
      LAND_SPEED = 0.5;    % 저고도 하강 속도 (m/s)
      LAND_CRAWL = 0.3;    % 극저속 하강 (m/s)

      if dist_to_ground > LAND_ALT1
          descent_speed = CRUISE_DN;
      elseif dist_to_ground > LAND_ALT2
          ratio = (dist_to_ground - LAND_ALT2) / (LAND_ALT1 - LAND_ALT2);
          descent_speed = LAND_SPEED + ratio * (CRUISE_DN - LAND_SPEED);
      elseif dist_to_ground > LAND_ALT3
          descent_speed = LAND_SPEED;
      else
          descent_speed = LAND_CRAWL;
      end
  end

== matlab function UAM_Flight_control/Flightmode/Auto/Guidance Mode Selector/GuidanceLogic.Land.Descend/MATLAB Function2 ==
  data: current_pos input; LAP output; descent_speed input
function LAP = calcLandLAP(current_pos, descent_speed)   
      persistent hold_n hold_e alt_cmd init_flag   
      dt = 0.005;                         
      if isempty(init_flag)
          hold_n = current_pos(1);
          hold_e = current_pos(2);                                                                                                                                                                                                                                     
          alt_cmd = current_pos(3);                                                                                                                                                                                                                                    
          init_flag = true;                                                                                                                                                                                                                                            
      end                                                                                                                                                                                                                                                   
                                                                                                                                                                                                                                                                       
      LAP = zeros(3, 1);                                                                                                                                                                                                                                               
      LAP(1) = hold_n;                                                                                                                                                                                                                                                 
      LAP(2) = hold_e;                                                                                                                                                                                                                                                 
                                                                                                                                                                                                                                                                       
      alt_cmd = alt_cmd + descent_speed * dt;                                                                                                                                                                                                                          
                                                                                                                                                                                                                                                                       
      % 현재 고도와 명령 고도 차이 제한 (최대 2m)                                                                                                                                                                                                                      
      if alt_cmd - current_pos(3) > 2.0                                                                                                                                                                                                                                
          alt_cmd = current_pos(3) + 2.0;                                                                                                                                                                                                                              
      end                                                                                                                                                                                                                                                              
                                                                                                                                                                                                                                                                       
      LAP(3) = alt_cmd;                                                                                                                                                                                                                                                
  end

== matlab function UAM_Flight_control/Flightmode/Auto/Guidance Mode Selector/GuidanceLogic.Land.Descend/MATLAB Function3 ==
  data: Pose3 input; LAD output; ToWP3 input
function LAD = calcLookahead(Pose3, ToWP3)
    AGL = ToWP3 - Pose3;
    if AGL > 50
        LAD = 10;
    elseif AGL > 30
        LAD = 5+(AGL - 10)/6;    % 5m→5, 10m→15
    elseif AGL > 15
        LAD = 1 + (AGL - 1)/6;    % 1m→1, 5m→5
    else
        LAD = max(0.5, AGL * 1);    % 최소 0.5
    end
  end

== matlab function UAM_Flight_control/Sensor/Subsystem1/MATLAB Function7 ==
  data: gps_h_msl input; z_gps_ned output; ref_valid output
function [z_gps_ned, ref_valid] = latch_gps_z_firstvalid(gps_h_msl)
%#codegen
% gps_h_msl : GNSS absolute altitude (m, Up+). Some systems output 0 when invalid.
% z_gps_ned : relative altitude in NED Down(+) [m] (up -> negative)
% ref_valid : reference latched?

persistent ref_set h_ref last_z
if isempty(ref_set)
    ref_set = false;
    h_ref   = 0.0;
    last_z  = 0.0;
end

% ---- define validity check ----
% Treat non-finite or near-zero as invalid (tune threshold if your system can be near sea level).
is_valid = isfinite(gps_h_msl) && (abs(gps_h_msl) > 1.0);

% ---- latch reference on first valid sample ----
if ~ref_set && is_valid
    h_ref   = gps_h_msl;
    ref_set = true;
end

% ---- output ----
if ref_set && is_valid
    z_gps_ned = -(gps_h_msl - h_ref);
    last_z    = z_gps_ned;   % optional: hold last good output
    ref_valid = true;
else
    % If reference not ready or GPS temporarily invalid:
    z_gps_ned = last_z;      % hold last value (or 0.0 if you prefer)
    ref_valid = ref_set;     % true if we already latched ref at least once
end
end
